simulink model "new_omega_simulink_verify"  (R2018a)
settings: Solver=VariableStepAuto  StartTime=0.0  StopTime=10  FixedStep=Ts  RelTol=1e-3
model workspace (MATLAB code in the model file):
  | m = 1500; cf = 19000; cr = 30000; lf = 1.2;
  | lr = 1.6; iz = 2500; v = 15;
  | 
  | A = [-(cf + cr)/(m * v), -(1 + (cf*lf - cr * lr)/(m * v^2));...
  |     -(cf*lf-cr*lr)/(iz), -(cf * lf^2 + cr + lr^2)/(iz * v)];
  | B = [cf/m/v;...
  |     cf*lf/iz];
  | C = [0 1];
  | D = 0;
  | 
  | ss1 = ss(A, B, C, D);
values from neighbouring files (symbols this model uses):
  Ap = [-2.58333333333  -0.957777777778; 6.08  -3.33653333333]    [all_current_space_0.mat]    (also in all_current_space_2.mat = [-7.75  -0.805; 3.12  -3.2496])
  Bp = [0.0844594594595 0.972972972973]    [all_current_space_0.mat]    (also in all_current_space_2.mat = [3.75 8.4])
  Cp = [0 1]    [all_current_space_0.mat]    (also in all_current_space_2.mat)
  Dp = 0    [all_current_space_0.mat]    (also in all_current_space_2.mat)
  KA = [0.99914515393  0.0277525115347  -0.00446849202581; -0.0277525115347  0.909546034947  0.146936049528; -0.00446849202582  -0.146936049528  0.724603883327]    [all_current_space_0.mat]    (also in all_current_space_2.mat; miu_controller.m = S.KA)
  KB = [0.00425809278186 0.0404673050461 0.0270400906943]    [all_current_space_0.mat]    (also in all_current_space_2.mat; miu_controller.m = S.KB)
  KC = [-0.0950993137051 0.986999497443 -0.879042893709]    [all_current_space_0.mat]    (also in all_current_space_2.mat; miu_controller.m = S.KC)
  KD = 0    [all_current_space_0.mat]    (also in all_current_space_2.mat; miu_controller.m = S.KD)
  Ts = 0.04    [all_current_space_0.mat]    (also in all_current_space_2.mat; limited_dynamic_0.m; limited_dynamic_1_main.m; main_matlab_script4.m)
libraries: simulink x1
settings Model: Creator=root  LastModifiedBy=root

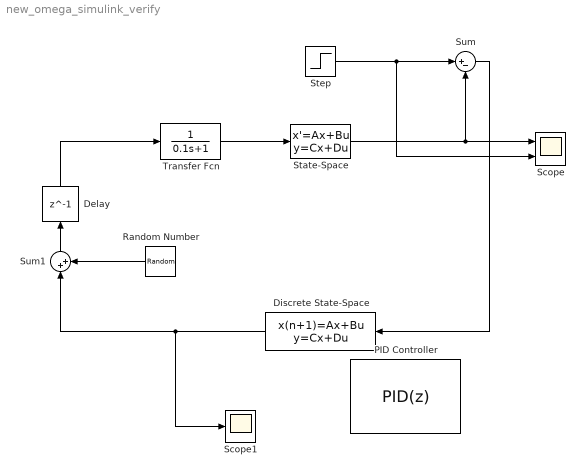
== system new_omega_simulink_verify ==
  Delay : Delay  DelayLength=1  SampleTime=Ts
  Discrete State-Space : DiscreteStateSpace  A=KA  B=KB  C=KC  D=KD  SampleTime=Ts
  PID Controller : simulink/Continuous/PID Controller  Controller=PID  TimeDomain=Discrete-time  SampleTime=Ts  IntegratorMethod=Forward Euler  FilterMethod=Forward Euler  Form=Parallel  UseFilter=off  ControllerParametersSource=internal  P=6.99547193941613  I=22.0442156288256  D=0.131091752536792  N=100  InitialConditionSource=internal  InitialConditionForIntegrator=0  InitialConditionForFilter=0  ExternalReset=none  LimitOutput=on  UpperSaturationLimit=4  LowerSaturationLimit=-4  LinearizeAsGain=on  AntiWindupMode=none  Kb=1  TrackingMode=off  Kt=1  SaturateOnIntegerOverflow=on  PParamMin=[]  PParamMax=[]  IParamMin=[]  IParamMax=[]  DParamMin=[]  DParamMax=[]  NParamMin=[]  NParamMax=[]  KbParamMin=[]  KbParamMax=[]  KtParamMin=[]  KtParamMax=[]  POutMin=[]  POutMax=[]  IOutMin=[]  IOutMax=[]  DOutMin=[]  DOutMax=[]  NOutMin=[]  NOutMax=[]  KbOutMin=[]  KbOutMax=[]  KtOutMin=[]  KtOutMax=[]  IntegratorOutMin=[]  IntegratorOutMax=[]  FilterOutMin=[]  FilterOutMax=[]  SumOutMin=[]  SumOutMax=[]  SumI1OutMin=[]  SumI1OutMax=[]  SumI2OutMin=[]  SumI2OutMax=[]  SumI3OutMin=[]  SumI3OutMax=[]  SumDOutMin=[]  SumDOutMax=[]  SaturationOutMin=[]  SaturationOutMax=[]  IntegratorContinuousStateAttributes=''  IntegratorStateMustResolveToSignalObject=off  IntegratorRTWStateStorageClass=Auto  FilterContinuousStateAttributes=''  FilterStateMustResolveToSignalObject=off  FilterRTWStateStorageClass=Auto  DifferentiatorICPrevScaledInput=0  DifferentiatorOutMin=[]  DifferentiatorOutMax=[]  FilterDiffOutCoefMin=[]  FilterDiffOutCoefMax=[]  SumDenOutMin=[]  SumDenOutMax=[]  SumNumOutMin=[]  SumNumOutMax=[]  ReciprocalOutMin=[]  ReciprocalOutMax=[]  DivideOutMin=[]  DivideOutMax=[]  TunerSelectOption=Transfer Function Based (PID Tuner App)
  Random Number : RandomNumber  Variance=0  SampleTime=Ts
  Scope : Scope  NumInputPorts=2
  Scope1 : Scope
  State-Space : StateSpace  A=Ap  B=Bp  C=Cp  D=Dp  InitialCondition=0
  Step : Step  Time=0.1  After=0.1  SampleTime=0
  Sum : Sum  Inputs=|+-
  Sum1 : Sum  Inputs=|++
  Transfer Fcn : TransferFcn  Denominator=[0.1 1]
  wires:
  Step/1 -> Scope/2, Sum/1
  State-Space/1 -> Sum/2, Scope/1
  Random Number/1 -> Sum1/2
  Sum1/1 -> Delay/1
  Delay/1 -> Transfer Fcn/1
  Transfer Fcn/1 -> State-Space/1
  Discrete State-Space/1 -> Scope1/1, Sum1/1
  Sum/1 -> Discrete State-Space/1
